simulink model "ysw_PID1"  (R2014a)
settings: Solver=ode45  StartTime=0.0  StopTime=10  RelTol=1e-3
values from neighbouring files (symbols this model uses):
  A = [  0 ,     1,                 0                 0 ... (first row only)    [ysw_PID.m]
  B = [0;  (I+m*l^2)/((M+m)*I+M*m*l^2);  0;  m*l/(((M+m)*I+M*m*l^2))]    [ysw_PID.m]
  C = [1 0 0 0;0 1 0 0;0 0 1 0;0 0 0 1]    [ysw_PID.m]
  D = [0;0;0;0]    [ysw_PID.m]
  K = place(A,B,p)    [ysw_PID.m]
settings Model: Creator=ii  LastModifiedBy=ii
settings SolverCC: ZeroCrossAlgorithm=Adaptive
settings DebuggingCC: UnderspecifiedInitializationDetection=Classic

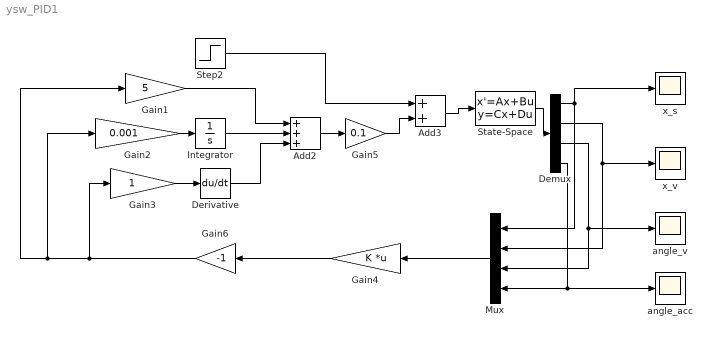
== system ysw_PID1 ==
  Add2 : Sum  Inputs=+++
  Add3 : Sum
  Demux : Demux
  Derivative : Derivative
  Gain1 : Gain  Gain=5
  Gain2 : Gain  Gain=0.001
  Gain3 : Gain
  Gain4 : Gain  Gain=K  Multiplication=Matrix(K*u)
  Gain5 : Gain  Gain=0.1
  Gain6 : Gain  Gain=-1
  Integrator : Integrator
  Mux : Mux
  State-Space : StateSpace  A=A  B=B  C=C  D=D  X0=0
  Step2 : Step  Time=0  SampleTime=0.01
  angle_acc : Scope
      settings: SaveName=ScopeData3
  angle_v : Scope
      settings: SaveName=ScopeData2
  x_s : Scope
  x_v : Scope
      settings: TimeRange=10
  wires:
  Step2/1 -> Add3/1
  State-Space/1 -> Demux/1
  Mux/1 -> Gain4/1
  Demux/1 -> Mux/1, x_s/1
  Demux/4 -> Mux/4, angle_acc/1
  Demux/3 -> Mux/3, angle_v/1
  Demux/2 -> x_v/1, Mux/2
  Gain1/1 -> Add2/1
  Gain2/1 -> Integrator/1
  Integrator/1 -> Add2/2
  Gain3/1 -> Derivative/1
  Derivative/1 -> Add2/3
  Add2/1 -> Gain5/1
  Add3/1 -> State-Space/1
  Gain5/1 -> Add3/2
  Gain4/1 -> Gain6/1
  Gain6/1 -> Gain3/1, Gain2/1, Gain1/1
